simulink model "PID_test_1_hydra"  (R2025b)
settings: Solver=FixedStepAuto  StartTime=0.0  StopTime=inf  RelTol=1e-3  EnableMultiTasking=on
undefined symbols (not defined in the file or in its folder): DiscIntNeverNeededParam
libraries: px4uORBlib x2, px4Sensorslib x2, simulink x1, sharedtransform x1, aerolibutil x1, px4Peripheralslib x1
settings Model: SimulationMode=external  ExtModeTrigDuration=10  Creator=lukas  LastModifiedBy=lukas
settings SolverCC: PositivePriorityOrder=on  AutoInsertRateTranBlk=on
settings OptimizationCC: EnhancedBackFolding=on  PassReuseOutputArgsAs=Individual arguments  ZeroExternalMemoryAtStartup=off  ZeroInternalMemoryAtStartup=off  MaxStackSize=64  OptimizeBlockOrder=speed  DifferentSizesBufferReuse=on  OptimizationCustomize=off  EfficientTunableParamExpr=on
settings DebuggingCC: MultiTaskRateTransMsg=warning  ParameterTunabilityLossMsg=error
settings HardwareCC: ProdBitPerPointer=32.0  ProdBitPerSizeT=32.0  ProdBitPerPtrDiffT=32.0  ProdLargestAtomicInteger=Long  ProdLargestAtomicFloat=Double  ProdWordSize=32.0  ProdLongLongMode=on  ProdHWDeviceType=ARM Compatible->ARM Cortex
settings SFSimCC: MATLABDynamicMemAlloc=off  SimTargetLang=C++  SimDLTargetLibrary=mkl-dnn
settings RTWCC: SystemTargetFile=ert.tlc  HardwareBoard=PX4 Host Target  TLCOptions="-aInlineSetEventsForThisBaseRateFcn=TLC_FALSE -aSuppressMultiTaskScheduler=TLC_FALSE  -aRateBasedStepFcn=0"  TemplateMakefile=ert_default_tmf  Toolchain=GNU Tools for PX4 Autopilots  PortableWordSizes=on  TargetLang=C++  Description=Embedded Coder
settings CodeAppCC: ForceParamTrailComments=on  IgnoreCustomStorageClasses=off  OperatorAnnotations=on  SimulinkDataObjDesc=on  SFDataObjDesc=on  InsertBlockDesc=on
settings ERTTargetCC: ExtModeTransport=2.0  ExtModeStaticAlloc=on  ExtModeMexFile=ext_xcp  ExtModeIntrfLevel=Level2 - Open  InlinedParameterPlacement=Hierarchical

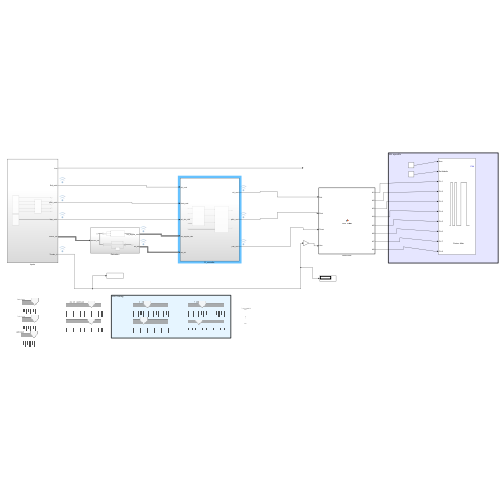
[thumbnail: Simulink's stored preview of the top-level diagram]
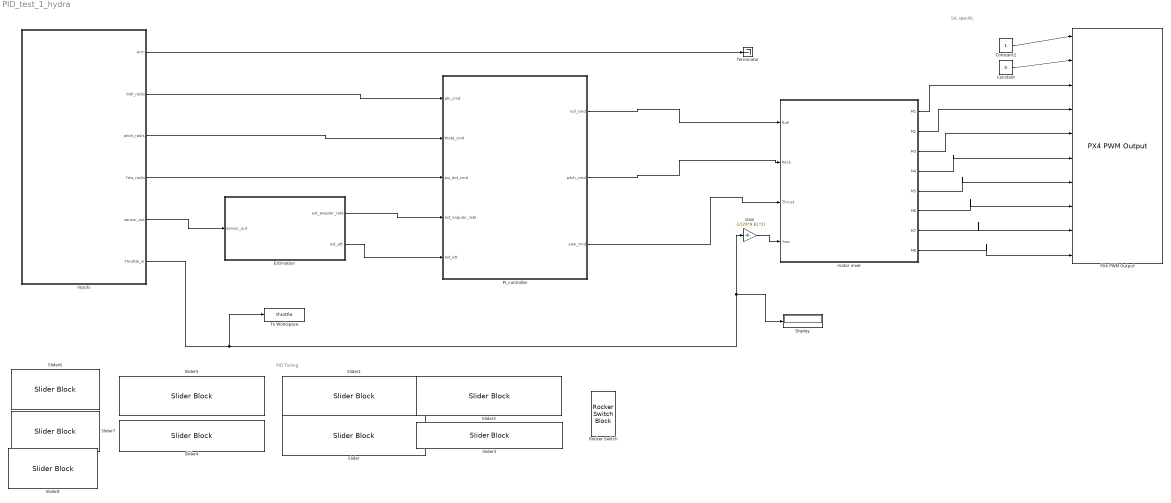
== system PID_test_1_hydra ==
  note: PID Tuning
  note: SIL specific
  Constant : Constant  Value=0  OutDataTypeStr=boolean
  Constant2 : Constant  OutDataTypeStr=boolean
  Display : Display
  Estimation : Subsystem
  Gain : Gain  Gain=-1/(20*9.81*2)
  Inputs : Subsystem
  "PI_controller " : Subsystem
  PX4 PWM Output : px4Peripheralslib/PX4 PWM Output  pwmDevice=Main  pwmChannel1_=on  pwmChannel2_=on  pwmChannel3_=on  pwmChannel4_=on  pwmChannel5_=on  pwmChannel6_=on  pwmChannel7_=on  pwmChannel8_=on
  Rocker Switch : RockerSwitchBlock
  Slider : SliderBlock  ScaleMax=0.1
  Slider1 : SliderBlock  ScaleMax=0.5
  Slider2 : SliderBlock  ScaleMax=0.5
  Slider3 : SliderBlock  ScaleMax=0.1
  Slider4 : SliderBlock  ScaleMax=1
  Slider5 : SliderBlock  ScaleMax=1
  Slider6 : SliderBlock  ScaleMax=4.5
  Slider7 : SliderBlock  ScaleMax=4.5
  Slider8 : SliderBlock  ScaleMax=4.5
  Terminator : Terminator
  To Workspace : ToWorkspace  VariableName=throttle  SaveFormat=Structure With Time  SampleTime=-1
  motor mxer : MATLAB Function  TreatAsAtomicUnit=on
  wires:
  "PI_controller "/2(pitch_cmd) -> motor mxer/2(Pitch)
  motor mxer/5(M5) -> PX4 PWM Output/7
  motor mxer/1(M1) -> PX4 PWM Output/3
  motor mxer/6(M6) -> PX4 PWM Output/8
  motor mxer/7(M7) -> PX4 PWM Output/9
  Constant/1 -> PX4 PWM Output/2
  motor mxer/3(M3) -> PX4 PWM Output/5
  Constant2/1 -> PX4 PWM Output/1
  Gain/1 -> motor mxer/4(Yaw)
  motor mxer/2(M2) -> PX4 PWM Output/4
  "PI_controller "/3(yaw_cmd) -> motor mxer/3(Thrust)
  Inputs/4(Yaw_rad/s) -> "PI_controller "/3(psi_dot_cmd)
  Inputs/1(Arm) -> Terminator/1
  Inputs/2(Roll_rad/s) -> "PI_controller "/1(phi_cmd)
  motor mxer/4(M4) -> PX4 PWM Output/6
  Inputs/6(Throttle_in) -> To Workspace/1, Gain/1, Display/1
  Inputs/3(pitch_rad/s) -> "PI_controller "/2(theta_cmd)
  motor mxer/8(M8) -> PX4 PWM Output/10
  Estimation/2(est_att) -> "PI_controller "/5(est_att)
  Inputs/5(sensor_out) -> Estimation/1(sensor_out)
  Estimation/1(est_angular_rate) -> "PI_controller "/4(est_angular_rate)
  "PI_controller "/1(roll_cmd) -> motor mxer/1(Roll)

== system PID_test_1_hydra/Estimation ==
  sensor_out : Inport
  Bus Creator : BusCreator  Inputs=3
  Bus Selector : BusSelector  OutputSignals=w_x_meas,w_y_meas,w_z_meas
  Bus Selector1 : BusSelector  OutputSignals=roll_meas,pitch_meas,yaw_meas
  MATLAB Function : MATLAB Function  TreatAsAtomicUnit=on
  Subsystem3 : Subsystem
  est_angular_rate : Outport
  est_att : Outport  Port=2
  wires:
  Subsystem3/1(est_angular_rate) -> est_angular_rate/1
  sensor_out/1 -> Bus Selector1/1, Bus Selector/1
  Bus Selector/1 -> Subsystem3/1(In1)  "<w_x_meas>"
  Bus Selector/2 -> Subsystem3/2(In2)  "<w_y_meas>"
  Bus Selector/3 -> Subsystem3/3(In3)  "<w_z_meas>"
  Bus Selector1/1 -> Bus Creator/1  "<roll_meas>"
  Bus Selector1/2 -> Bus Creator/2  "<pitch_meas>"
  Bus Selector1/3 -> MATLAB Function/1(yaw_w)  "<yaw_meas>"
  Bus Creator/1 -> est_att/1
  MATLAB Function/1(yaw_u) -> Bus Creator/3  "yaw"

== system PID_test_1_hydra/Inputs ==
  RC_input : Subsystem
  Sensors_meas : Subsystem
  Stick_mapping : Subsystem
  Arm : Outport
  Roll_rad/s : Outport  Port=2
  pitch_rad/s : Outport  Port=3
  Yaw_rad/s : Outport  Port=4
  sensor_out : Outport  Port=5
  Throttle_in : Outport  Port=6
  wires:
  Sensors_meas/1(sensor_out) -> sensor_out/1
  RC_input/1(Arm) -> Arm/1
  RC_input/2(Roll_in) -> Stick_mapping/1(Roll_in)
  RC_input/3(Pitch_in) -> Stick_mapping/2(Pitch_in)
  RC_input/4(Throttle_in) -> Stick_mapping/3(Throttle_in)
  RC_input/5(Yaw_in) -> Stick_mapping/4(yaw_in)
  Stick_mapping/1(Roll_rad) -> Roll_rad/s/1
  Stick_mapping/2(Pitch_rad) -> pitch_rad/s/1
  Stick_mapping/3(Throttle) -> Throttle_in/1
  Stick_mapping/4(yaw_rad/s) -> Yaw_rad/s/1

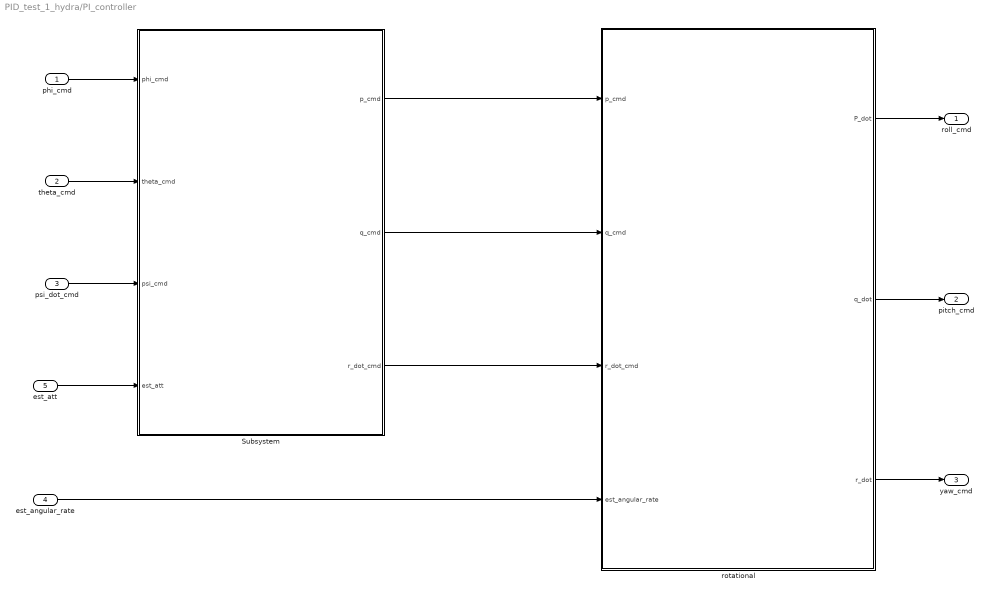
== system PID_test_1_hydra/PI_controller  ==
  phi_cmd : Inport
  theta_cmd : Inport  Port=2
  psi_dot_cmd : Inport  Port=3
  est_angular_rate : Inport  Port=4
  est_att : Inport  Port=5
  Subsystem : Subsystem
  rotational : Subsystem
  roll_cmd : Outport
  pitch_cmd : Outport  Port=2
  yaw_cmd : Outport  Port=3
  wires:
  phi_cmd/1 -> Subsystem/1(phi_cmd)
  theta_cmd/1 -> Subsystem/2(theta_cmd)
  psi_dot_cmd/1 -> Subsystem/3(psi_cmd)
  est_att/1 -> Subsystem/4(est_att)
  est_angular_rate/1 -> rotational/4(est_angular_rate)
  Subsystem/1(p_cmd) -> rotational/1(p_cmd)
  Subsystem/2(q_cmd) -> rotational/2(q_cmd)
  Subsystem/3(r_dot_cmd) -> rotational/3(r_dot_cmd)
  rotational/1(P_dot) -> roll_cmd/1
  rotational/2(q_dot) -> pitch_cmd/1
  rotational/3(r_dot) -> yaw_cmd/1

== system PID_test_1_hydra/Estimation/Subsystem3 ==
  In1 : Inport
  In2 : Inport  Port=2
  In3 : Inport  Port=3
  Bus Creator : BusCreator  Inputs=3
  Subsystem : Subsystem
  Subsystem1 : Subsystem
  Subsystem2 : Subsystem
  est_angular_rate : Outport
  wires:
  Bus Creator/1 -> est_angular_rate/1
  Subsystem/1(Out1) -> Bus Creator/1  "est_p"
  In3/1 -> Subsystem2/1(In1)
  In2/1 -> Subsystem1/1(In1)
  Subsystem2/1(Out1) -> Bus Creator/3  "est_r"
  Subsystem1/1(Out1) -> Bus Creator/2  "est_q"
  In1/1 -> Subsystem/1(In1)

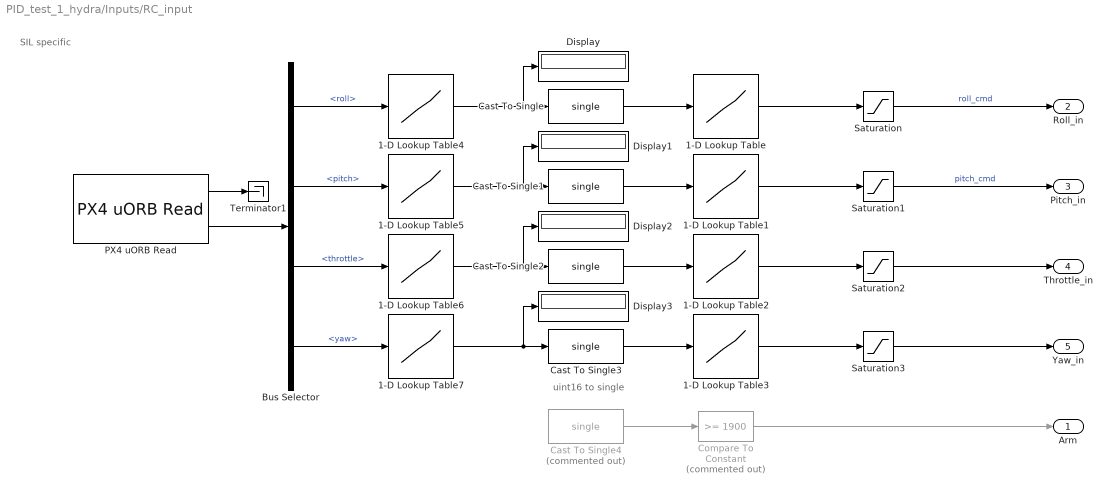
== system PID_test_1_hydra/Inputs/RC_input ==
  note: uint16 to single
  note: SIL specific
  1-D Lookup Table : Lookup_n-D  NumberOfTableDimensions=1  BreakpointsForDimension1=([1000 1500 2000])  Table=single([-1 0 1])  InternalRulePriority=Speed  RndMeth=Simplest
  1-D Lookup Table1 : Lookup_n-D  NumberOfTableDimensions=1  BreakpointsForDimension1=([1000 1500 2000])  Table=single([-1 0 1])  InternalRulePriority=Speed  RndMeth=Simplest
  1-D Lookup Table2 : Lookup_n-D  NumberOfTableDimensions=1  BreakpointsForDimension1=([1000 1500 2000])  Table=single([0 0.5 1])  InternalRulePriority=Speed  RndMeth=Simplest
  1-D Lookup Table3 : Lookup_n-D  NumberOfTableDimensions=1  BreakpointsForDimension1=([1000 1500 2000])  Table=single([-1 0 1])  InternalRulePriority=Speed  RndMeth=Simplest
  1-D Lookup Table4 : Lookup_n-D  NumberOfTableDimensions=1  BreakpointsForDimension1=[-1, 0,1]  Table=single([1000, 1500, 2000])  InternalRulePriority=Speed  RndMeth=Simplest
  1-D Lookup Table5 : Lookup_n-D  NumberOfTableDimensions=1  BreakpointsForDimension1=[-1, 0,1]  Table=single([1000, 1500, 2000])  InternalRulePriority=Speed  RndMeth=Simplest
  1-D Lookup Table6 : Lookup_n-D  NumberOfTableDimensions=1  BreakpointsForDimension1=[0,1]  Table="single([1000,  2000])"  InternalRulePriority=Speed  RndMeth=Simplest
  1-D Lookup Table7 : Lookup_n-D  NumberOfTableDimensions=1  BreakpointsForDimension1=[-1, 0,1]  Table=single([1000, 1500, 2000])  InternalRulePriority=Speed  RndMeth=Simplest
  Bus Selector : BusSelector  OutputSignals=roll,pitch,throttle,yaw
  Cast To Single{,1..3} (4 alike) : DataTypeConversion  OutDataTypeStr=single  SaturateOnIntegerOverflow=off  RndMeth=Floor
  Cast To Single4 : DataTypeConversion  Commented=on  OutDataTypeStr=single  SaturateOnIntegerOverflow=off  RndMeth=Floor
  Compare To Constant : simulink/Logic and Bit Operations/Compare To Constant  Commented=on  relop=>=  const=1900  OutDataTypeStr=boolean
  Display{,1..3} (4 alike) : Display
  PX4 uORB Read : px4uORBlib/PX4 uORB Read  uORBTopic=ManualControlSetpoint  selectInstance=manual_control_setpoint  SampleTime=0.001  BlockingMode=off  BlockTimeout=1e-3
  Saturation : Saturate  UpperLimit=1  LowerLimit=-1
  Saturation1 : Saturate  UpperLimit=1  LowerLimit=-1
  Saturation2 : Saturate  UpperLimit=1  LowerLimit=0
  Saturation3 : Saturate  UpperLimit=1  LowerLimit=-1
  Terminator1 : Terminator
  Arm : Outport
  Roll_in : Outport  Port=2
  Pitch_in : Outport  Port=3
  Throttle_in : Outport  Port=4
  Yaw_in : Outport  Port=5
  wires:
  Compare To Constant/1 -> Arm/1
  Bus Selector/3 -> 1-D Lookup Table6/1  "<throttle>"
  Saturation3/1 -> Yaw_in/1
  Cast To Single/1 -> 1-D Lookup Table/1
  Saturation2/1 -> Throttle_in/1
  Bus Selector/2 -> 1-D Lookup Table5/1  "<pitch>"
  Cast To Single1/1 -> 1-D Lookup Table1/1
  Cast To Single3/1 -> 1-D Lookup Table3/1
  Cast To Single4/1 -> Compare To Constant/1
  Cast To Single2/1 -> 1-D Lookup Table2/1
  Saturation1/1 -> Pitch_in/1  "pitch_cmd"
  Saturation/1 -> Roll_in/1  "roll_cmd"
  1-D Lookup Table/1 -> Saturation/1
  1-D Lookup Table1/1 -> Saturation1/1
  1-D Lookup Table2/1 -> Saturation2/1
  1-D Lookup Table3/1 -> Saturation3/1
  Bus Selector/4 -> 1-D Lookup Table7/1  "<yaw>"
  Bus Selector/1 -> 1-D Lookup Table4/1  "<roll>"
  PX4 uORB Read/2 -> Bus Selector/1
  PX4 uORB Read/1 -> Terminator1/1
  1-D Lookup Table4/1 -> Display/1, Cast To Single/1
  1-D Lookup Table5/1 -> Display1/1, Cast To Single1/1
  1-D Lookup Table7/1 -> Display3/1, Cast To Single3/1
  1-D Lookup Table6/1 -> Display2/1, Cast To Single2/1

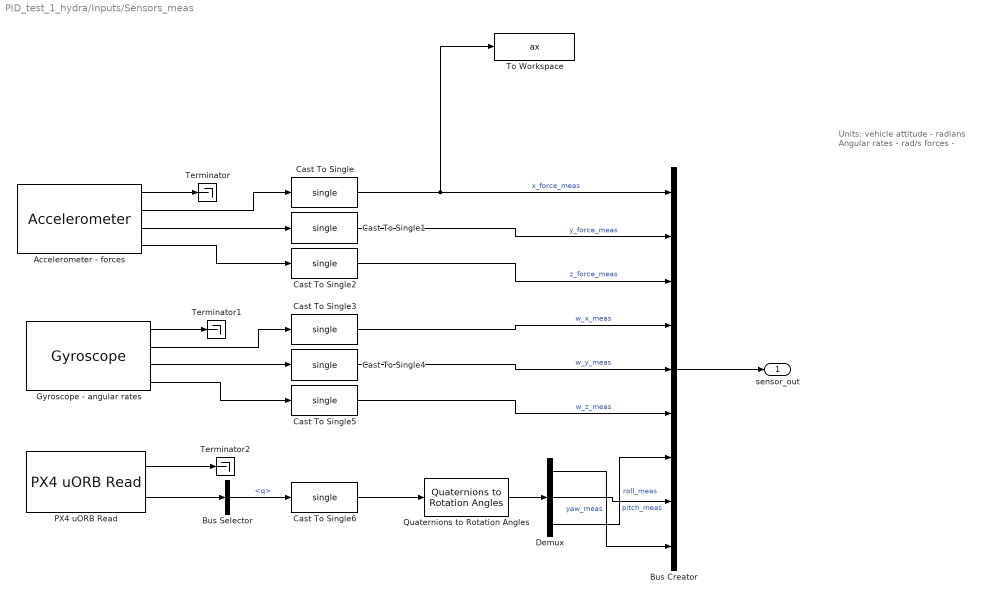
== system PID_test_1_hydra/Inputs/Sensors_meas ==
  note: Units:
      | vehicle attitude - radians
      | Angular rates - rad/s
      | forces -
  "Accelerometer - forces " : px4Sensorslib/Accelerometer  uorbTimeStamp=off  BlockingMode=off  BlockTimeout=1e-3  sampleTime=1/250
  Bus Creator : BusCreator  Inputs=9
  Bus Selector : BusSelector  OutputSignals=q
  Cast To Single{,1..6} (7 alike) : DataTypeConversion  OutDataTypeStr=single  SaturateOnIntegerOverflow=off  RndMeth=Floor
  Demux : Demux  Outputs=3
  Gyroscope - angular rates : px4Sensorslib/Gyroscope  uorbTimeStamp=off  BlockingMode=off  BlockTimeout=1e-3  sampleTime=1/250
  PX4 uORB Read : px4uORBlib/PX4 uORB Read  uORBTopic=VehicleAttitude  selectInstance=vehicle_attitude  SampleTime=-1  BlockingMode=off  BlockTimeout=1e-3
  Quaternions to Rotation Angles : sharedtransform/Quaternions to Rotation Angles  rotationOrder=ZYX  aMode=aMode
  Terminator : Terminator
  Terminator1 : Terminator
  Terminator2 : Terminator
  To Workspace : ToWorkspace  VariableName=ax  SaveFormat=Structure With Time  SampleTime=-1
  sensor_out : Outport
  wires:
  PX4 uORB Read/1 -> Terminator2/1
  Gyroscope - angular rates/1 -> Terminator1/1
  Cast To Single4/1 -> Bus Creator/5  "w_y_meas"
  Gyroscope - angular rates/2 -> Cast To Single3/1
  "Accelerometer - forces "/1 -> Terminator/1
  Demux/3 -> Bus Creator/7  "roll_meas"
  Demux/2 -> Bus Creator/8  "pitch_meas"
  Demux/1 -> Bus Creator/9  "yaw_meas"
  Gyroscope - angular rates/3 -> Cast To Single4/1
  Gyroscope - angular rates/4 -> Cast To Single5/1
  Cast To Single5/1 -> Bus Creator/6  "w_z_meas"
  Bus Creator/1 -> sensor_out/1
  "Accelerometer - forces "/2 -> Cast To Single/1
  Bus Selector/1 -> Cast To Single6/1  "<q>"
  "Accelerometer - forces "/3 -> Cast To Single1/1
  Cast To Single/1 -> To Workspace/1, Bus Creator/1  "x_force_meas"
  PX4 uORB Read/2 -> Bus Selector/1
  "Accelerometer - forces "/4 -> Cast To Single2/1
  Cast To Single6/1 -> Quaternions to Rotation Angles/1
  Quaternions to Rotation Angles/1 -> Demux/1
  Cast To Single3/1 -> Bus Creator/4  "w_x_meas"
  Cast To Single1/1 -> Bus Creator/2  "y_force_meas"
  Cast To Single2/1 -> Bus Creator/3  "z_force_meas"

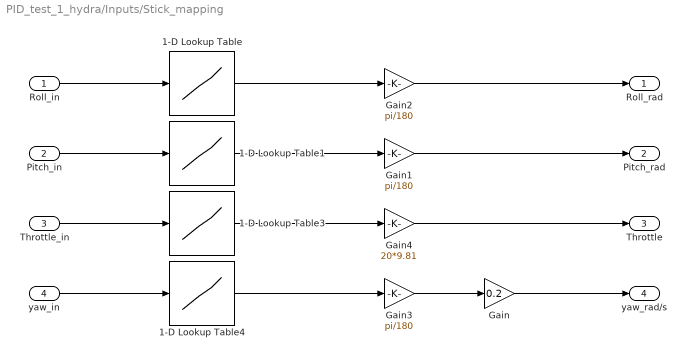
== system PID_test_1_hydra/Inputs/Stick_mapping ==
  Roll_in : Inport
  Pitch_in : Inport  Port=2
  Throttle_in : Inport  Port=3
  yaw_in : Inport  Port=4
  1-D Lookup Table : Lookup_n-D  NumberOfTableDimensions=1  BreakpointsForDimension1=single([-1,1])  Table=single([-30,30])  InternalRulePriority=Speed  RndMeth=Simplest
  1-D Lookup Table1 : Lookup_n-D  NumberOfTableDimensions=1  BreakpointsForDimension1=single([-1,1])  Table=single([30,-30])  InternalRulePriority=Speed  RndMeth=Simplest
  1-D Lookup Table3 : Lookup_n-D  NumberOfTableDimensions=1  BreakpointsForDimension1=single([0 0.100000001 0.25 0.5 0.75 1])  Table=single([0 -0.200000003 -0.5 -1 -1.5 -2])  InternalRulePriority=Speed  RndMeth=Simplest
  1-D Lookup Table4 : Lookup_n-D  NumberOfTableDimensions=1  BreakpointsForDimension1=single([-1,1])  Table=single([-90,90])  InternalRulePriority=Speed  RndMeth=Simplest
  Gain : Gain  Gain=0.2
  Gain1 : Gain  Gain=pi/180
  Gain2 : Gain  Gain=pi/180
  Gain3 : Gain  Gain=pi/180
  Gain4 : Gain  Gain=20*9.81
  Roll_rad : Outport
  Pitch_rad : Outport  Port=2
  Throttle : Outport  Port=3
  yaw_rad/s : Outport  Port=4
  wires:
  Gain1/1 -> Pitch_rad/1
  Roll_in/1 -> 1-D Lookup Table/1
  Pitch_in/1 -> 1-D Lookup Table1/1
  yaw_in/1 -> 1-D Lookup Table4/1
  Throttle_in/1 -> 1-D Lookup Table3/1
  1-D Lookup Table1/1 -> Gain1/1
  1-D Lookup Table/1 -> Gain2/1
  1-D Lookup Table3/1 -> Gain4/1
  1-D Lookup Table4/1 -> Gain3/1
  Gain2/1 -> Roll_rad/1
  Gain3/1 -> Gain/1
  Gain4/1 -> Throttle/1
  Gain/1 -> yaw_rad/s/1

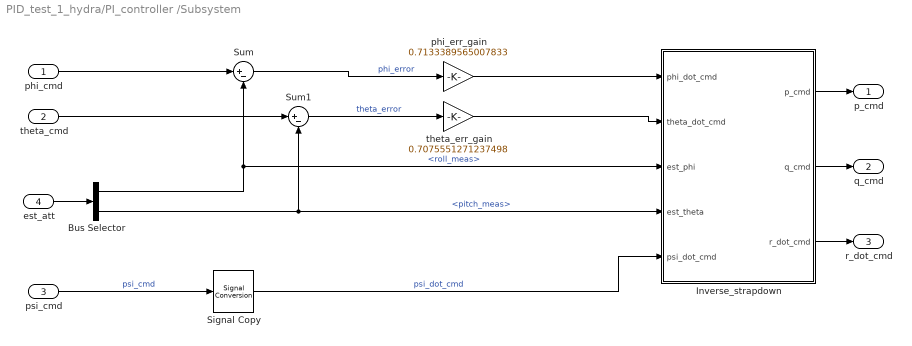
== system PID_test_1_hydra/PI_controller /Subsystem ==
  phi_cmd : Inport
  theta_cmd : Inport  Port=2
  psi_cmd : Inport  Port=3
  est_att : Inport  Port=4
  Bus Selector : BusSelector  OutputSignals=roll_meas,pitch_meas
  Inverse_strapdown : Subsystem
  Signal Copy : SignalConversion  OverrideOpt=off
  Sum : Sum  Inputs=|+-
  Sum1 : Sum  Inputs=|+-
  phi_err_gain : Gain  Gain=0.7133389565007833
  theta_err_gain : Gain  Gain=0.7075551271237498
  p_cmd : Outport
  q_cmd : Outport  Port=2
  r_dot_cmd : Outport  Port=3
  wires:
  Bus Selector/2 -> Inverse_strapdown/4(est_theta), Sum1/2  "<pitch_meas>"
  Bus Selector/1 -> Inverse_strapdown/3(est_phi), Sum/2  "<roll_meas>"
  Sum1/1 -> theta_err_gain/1  "theta_error"
  theta_cmd/1 -> Sum1/1
  phi_cmd/1 -> Sum/1
  Sum/1 -> phi_err_gain/1  "phi_error"
  psi_cmd/1 -> Signal Copy/1  "psi_cmd"
  Signal Copy/1 -> Inverse_strapdown/5(psi_dot_cmd)  "psi_dot_cmd"
  est_att/1 -> Bus Selector/1
  phi_err_gain/1 -> Inverse_strapdown/1(phi_dot_cmd)
  theta_err_gain/1 -> Inverse_strapdown/2(theta_dot_cmd)
  Inverse_strapdown/1(p_cmd) -> p_cmd/1
  Inverse_strapdown/2(q_cmd) -> q_cmd/1
  Inverse_strapdown/3(r_dot_cmd) -> r_dot_cmd/1

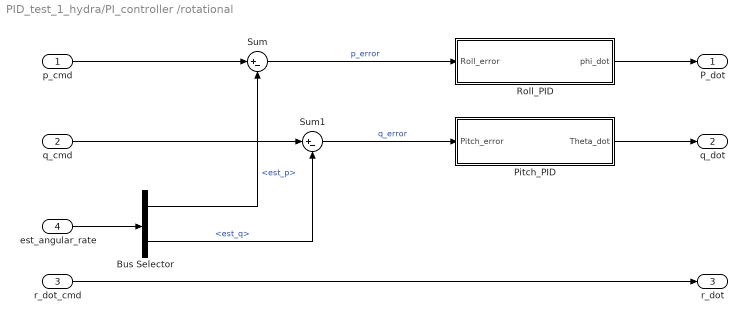
== system PID_test_1_hydra/PI_controller /rotational ==
  p_cmd : Inport
  q_cmd : Inport  Port=2
  r_dot_cmd : Inport  Port=3
  est_angular_rate : Inport  Port=4
  Bus Selector : BusSelector  OutputSignals=est_p,est_q
  Pitch_PID : Subsystem
  Roll_PID : Subsystem
  Sum : Sum  Inputs=|+-
  Sum1 : Sum  Inputs=|+-
  P_dot : Outport
  q_dot : Outport  Port=2
  r_dot : Outport  Port=3
  wires:
  Sum/1 -> Roll_PID/1(Roll_error)  "p_error"
  Sum1/1 -> Pitch_PID/1(Pitch_error)  "q_error"
  Roll_PID/1(phi_dot) -> P_dot/1
  Bus Selector/2 -> Sum1/2  "<est_q>"
  p_cmd/1 -> Sum/1
  Pitch_PID/1(Theta_dot) -> q_dot/1
  r_dot_cmd/1 -> r_dot/1
  q_cmd/1 -> Sum1/1
  Bus Selector/1 -> Sum/2  "<est_p>"
  est_angular_rate/1 -> Bus Selector/1

== system PID_test_1_hydra/Estimation/Subsystem3/Subsystem ==
  In1 : Inport
  DI : Subsystem
  Gain : Gain  Gain=single(4.5)
  Saturation1 : Saturate  UpperLimit=5.24  LowerLimit=-5.24
  Sum : Sum  Inputs=|+-
  Out1 : Outport
  wires:
  Sum/1 -> Gain/1
  Gain/1 -> DI/1(In1)
  DI/1(Out1) -> Saturation1/1, Sum/2
  In1/1 -> DI/2(In2), Sum/1
  Saturation1/1 -> Out1/1

== system PID_test_1_hydra/Estimation/Subsystem3/Subsystem1 ==
  In1 : Inport
  DI : Subsystem
  Gain : Gain  Gain=4.5
  Saturation1 : Saturate  UpperLimit=5.24  LowerLimit=-5.24
  Sum : Sum  Inputs=|+-
  Out1 : Outport
  wires:
  Sum/1 -> Gain/1
  DI/1(Out1) -> Saturation1/1, Sum/2
  Gain/1 -> DI/1(In1)
  In1/1 -> DI/2(In2), Sum/1
  Saturation1/1 -> Out1/1

== system PID_test_1_hydra/Estimation/Subsystem3/Subsystem2 ==
  In1 : Inport
  DI : Subsystem
  Gain : Gain  Gain=4.5
  Saturation1 : Saturate  UpperLimit=5.24  LowerLimit=-5.24
  Sum : Sum  Inputs=|+-
  Out1 : Outport
  wires:
  Sum/1 -> Gain/1
  DI/1(Out1) -> Saturation1/1, Sum/2
  Gain/1 -> DI/1(In1)
  In1/1 -> DI/2(In2), Sum/1
  Saturation1/1 -> Out1/1

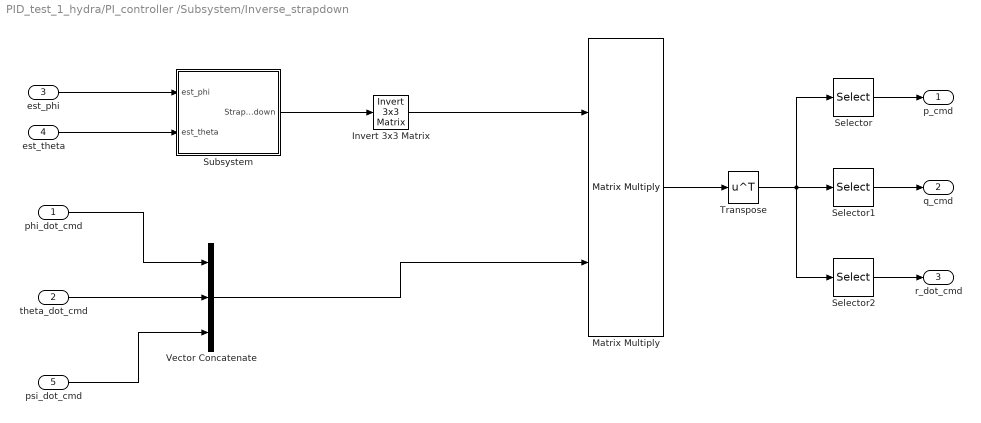
== system PID_test_1_hydra/PI_controller /Subsystem/Inverse_strapdown ==
  phi_dot_cmd : Inport
  theta_dot_cmd : Inport  Port=2
  est_phi : Inport  Port=3
  est_theta : Inport  Port=4
  psi_dot_cmd : Inport  Port=5
  Invert 3x3 Matrix : aerolibutil/Invert  3x3 Matrix
  Matrix Multiply : Product  Multiplication=Matrix(*)
  Selector : Selector  InputPortWidth=3  IndexOptions=Index vector (dialog)  Indices=1  OutputSizes=1
  Selector1 : Selector  InputPortWidth=3  IndexOptions=Index vector (dialog)  Indices=2  OutputSizes=1
  Selector2 : Selector  InputPortWidth=3  IndexOptions=Index vector (dialog)  Indices=3  OutputSizes=1
  Subsystem : Subsystem
  Transpose : Math  Operator=transpose
  Vector Concatenate : Concatenate  NumInputs=3  Mode=Multidimensional array
  p_cmd : Outport
  q_cmd : Outport  Port=2
  r_dot_cmd : Outport  Port=3
  wires:
  Vector Concatenate/1 -> Matrix Multiply/2
  Subsystem/1(Strap_down) -> Invert 3x3 Matrix/1
  Invert 3x3 Matrix/1 -> Matrix Multiply/1
  est_phi/1 -> Subsystem/1(est_phi)
  est_theta/1 -> Subsystem/2(est_theta)
  Matrix Multiply/1 -> Transpose/1
  Transpose/1 -> Selector2/1, Selector1/1, Selector/1
  Selector/1 -> p_cmd/1
  Selector1/1 -> q_cmd/1
  Selector2/1 -> r_dot_cmd/1
  phi_dot_cmd/1 -> Vector Concatenate/1
  theta_dot_cmd/1 -> Vector Concatenate/2
  psi_dot_cmd/1 -> Vector Concatenate/3

== system PID_test_1_hydra/PI_controller /rotational/Pitch_PID ==
  Pitch_error : Inport
  Discrete-Time Integrator : DiscreteIntegrator  SampleTime=-1  ICPrevOutput=DiscIntNeverNeededParam  ICPrevScaledInput=DiscIntNeverNeededParam
  I_pitch : Gain  Gain=single(0.02936526)
  P_pitch : Gain  Gain=0.2
  Sum : Sum  Inputs=|++
  Theta_dot : Outport
  wires:
  Sum/1 -> Theta_dot/1
  Discrete-Time Integrator/1 -> I_pitch/1
  P_pitch/1 -> Sum/1
  Pitch_error/1 -> Discrete-Time Integrator/1, P_pitch/1
  I_pitch/1 -> Sum/2

== system PID_test_1_hydra/PI_controller /rotational/Roll_PID ==
  Roll_error : Inport
  Discrete-Time Integrator : DiscreteIntegrator  gainval=1  SampleTime=-1  ICPrevOutput=DiscIntNeverNeededParam  ICPrevScaledInput=DiscIntNeverNeededParam
  I_roll : Gain  Gain=0.03033785294146734
  P_roll : Gain  Gain=0.2
  Sum : Sum  Inputs=|++
  phi_dot : Outport
  wires:
  Sum/1 -> phi_dot/1
  P_roll/1 -> Sum/1
  I_roll/1 -> Discrete-Time Integrator/1  "int_err_unsat"
  Discrete-Time Integrator/1 -> Sum/2
  Roll_error/1 -> I_roll/1, P_roll/1

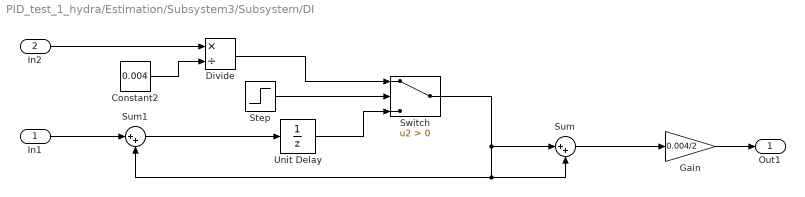
== system PID_test_1_hydra/Estimation/Subsystem3/Subsystem/DI ==
  In1 : Inport
  In2 : Inport  Port=2
  Constant2 : Constant  Value=0.004
  Divide : Product  Inputs=*/
  Gain : Gain  Gain=0.004/2
  Step : Step  Time=0.02  Before=1  After=0  SampleTime=0.004
  Sum : Sum  Inputs=|++
  Sum1 : Sum  Inputs=|++
  Switch : Switch  Criteria=u2 > Threshold  SaturateOnIntegerOverflow=off  InputSameDT=off
  Unit Delay : UnitDelay  SampleTime=-1  HasFrameUpgradeWarning=on
  Out1 : Outport
  wires:
  Step/1 -> Switch/2
  Sum1/1 -> Unit Delay/1
  Unit Delay/1 -> Switch/3
  Divide/1 -> Switch/1
  Switch/1 -> Sum1/2, Sum/2, Sum/1
  Sum/1 -> Gain/1
  Constant2/1 -> Divide/2
  Gain/1 -> Out1/1
  In1/1 -> Sum1/1
  In2/1 -> Divide/1

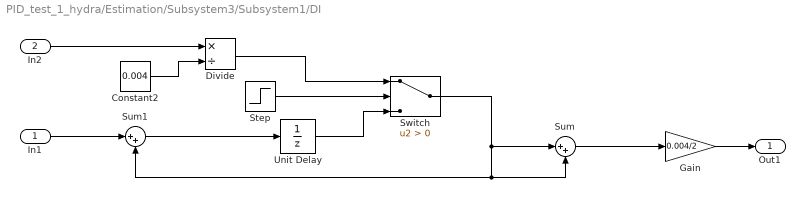
== system PID_test_1_hydra/Estimation/Subsystem3/Subsystem1/DI ==
  In1 : Inport
  In2 : Inport  Port=2
  Constant2 : Constant  Value=0.004
  Divide : Product  Inputs=*/
  Gain : Gain  Gain=0.004/2
  Step : Step  Time=0.02  Before=1  After=0  SampleTime=0.004
  Sum : Sum  Inputs=|++
  Sum1 : Sum  Inputs=|++
  Switch : Switch  Criteria=u2 > Threshold  SaturateOnIntegerOverflow=off  InputSameDT=off
  Unit Delay : UnitDelay  SampleTime=-1  HasFrameUpgradeWarning=on
  Out1 : Outport
  wires:
  Step/1 -> Switch/2
  Sum1/1 -> Unit Delay/1
  Unit Delay/1 -> Switch/3
  Divide/1 -> Switch/1
  Switch/1 -> Sum1/2, Sum/2, Sum/1
  Sum/1 -> Gain/1
  Constant2/1 -> Divide/2
  Gain/1 -> Out1/1
  In1/1 -> Sum1/1
  In2/1 -> Divide/1

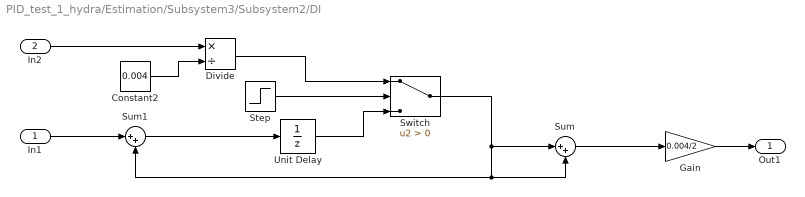
== system PID_test_1_hydra/Estimation/Subsystem3/Subsystem2/DI ==
  In1 : Inport
  In2 : Inport  Port=2
  Constant2 : Constant  Value=0.004
  Divide : Product  Inputs=*/
  Gain : Gain  Gain=0.004/2
  Step : Step  Time=0.02  Before=1  After=0  SampleTime=0.004
  Sum : Sum  Inputs=|++
  Sum1 : Sum  Inputs=|++
  Switch : Switch  Criteria=u2 > Threshold  SaturateOnIntegerOverflow=off  InputSameDT=off
  Unit Delay : UnitDelay  SampleTime=-1  HasFrameUpgradeWarning=on
  Out1 : Outport
  wires:
  Step/1 -> Switch/2
  Sum1/1 -> Unit Delay/1
  Unit Delay/1 -> Switch/3
  Divide/1 -> Switch/1
  Switch/1 -> Sum1/2, Sum/2, Sum/1
  Sum/1 -> Gain/1
  Constant2/1 -> Divide/2
  Gain/1 -> Out1/1
  In1/1 -> Sum1/1
  In2/1 -> Divide/1

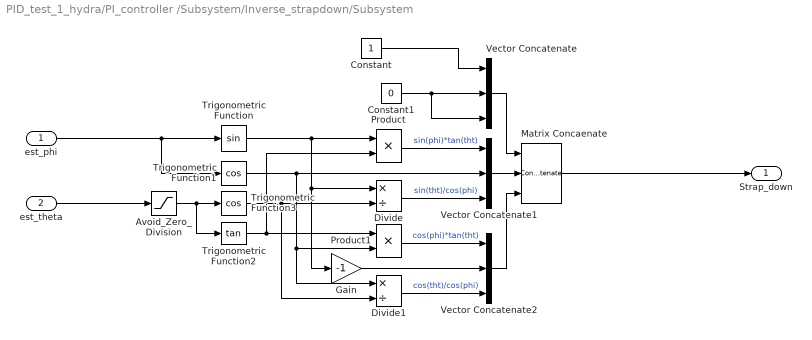
== system PID_test_1_hydra/PI_controller /Subsystem/Inverse_strapdown/Subsystem ==
  est_phi : Inport
  est_theta : Inport  Port=2
  Avoid_Zero_Division : Saturate  UpperLimit=pi/2*0.9  LowerLimit=-pi/2*0.9
  Constant : Constant  OutDataTypeStr=single
  Constant1 : Constant  Value=0  OutDataTypeStr=single
  Divide : Product  Inputs=*/
  Divide1 : Product  Inputs=*/
  Gain : Gain  Gain=-1
  Matrix Concaenate : Concatenate  NumInputs=3  Mode=Multidimensional array  ConcatenateDimension=2
  Product : Product  RndMeth=Zero
  Product1 : Product  RndMeth=Zero
  Trigonometric Function : Trigonometry
  Trigonometric Function1 : Trigonometry  Operator=cos
  Trigonometric Function2 : Trigonometry  Operator=tan
  Trigonometric Function3 : Trigonometry  Operator=cos
  Vector Concatenate : Concatenate  NumInputs=3  Mode=Multidimensional array
  Vector Concatenate1 : Concatenate  NumInputs=3  Mode=Multidimensional array
  Vector Concatenate2 : Concatenate  NumInputs=3  Mode=Multidimensional array
  Strap_down : Outport
  wires:
  Vector Concatenate1/1 -> Matrix Concaenate/2
  Product1/1 -> Vector Concatenate2/1  "cos(phi)*tan(tht)"
  Trigonometric Function1/1 -> Vector Concatenate1/2, Divide1/1, Product1/2
  est_phi/1 -> Trigonometric Function1/1, Trigonometric Function/1
  Constant1/1 -> Vector Concatenate/2, Vector Concatenate/3
  Trigonometric Function3/1 -> Divide/2, Divide1/2
  Avoid_Zero_Division/1 -> Trigonometric Function3/1, Trigonometric Function2/1
  Gain/1 -> Vector Concatenate2/2
  Divide/1 -> Vector Concatenate1/3  "sin(tht)/cos(phi)"
  Vector Concatenate2/1 -> Matrix Concaenate/3
  Divide1/1 -> Vector Concatenate2/3  "cos(tht)/cos(phi)"
  est_theta/1 -> Avoid_Zero_Division/1
  Product/1 -> Vector Concatenate1/1  "sin(phi)*tan(tht)"
  Vector Concatenate/1 -> Matrix Concaenate/1
  Constant/1 -> Vector Concatenate/1
  Matrix Concaenate/1 -> Strap_down/1
  Trigonometric Function2/1 -> Product/2, Product1/1
  Trigonometric Function/1 -> Product/1, Divide/1, Gain/1

== matlab function PID_test_1_hydra/motor mxer ==
  data: Roll input; M1 output; Pitch input; Thrust input; Yaw input; M2 output; M3 output; M4 output; M5 output; M6 output; M7 output; M8 output
function [M1, M2, M3, M4, M5, M6, M7, M8] = motor_mixer(Roll, Pitch, Thrust, Yaw)
% This function calculates motor commands for the 8-motor "plus" 
% configuration shown in your image.
%
% Inputs (assumed):
%   Roll, Pitch, Yaw: -1.0 to +1.0 control inputs
%   Thrust:             0.0 to 1.0 base throttle

% --- Configuration ---
idle_PWM = uint16(1000);
max_motor_val = single(1.0); % Max normalized output
min_motor_val = single(0.0); % Min normalized output

% This scaling method is from your example. It scales the control 
% inputs by the thrust level. You may need to tune the '4.0'
% denominator for best performance.
control_scale = Thrust / single(4.0);

% --- Mixer Logic ---
% Calculate normalized motor values (0.0 to 1.0 range) based on the diagram.
% We use single() to ensure floating-point math, as in your example.

% M1 (Front, CCW): -Pitch, +Yaw
m1_norm = ( ( -Pitch + Yaw ) * control_scale + Thrust );

% M2 (Back, CCW): +Pitch, +Yaw
m2_norm = ( (  Pitch + Yaw ) * control_scale + Thrust );

% M3 (Front-Right, CW): -Pitch, -Roll, -Yaw
m3_norm = ( ( -Pitch - Roll - Yaw ) * control_scale + Thrust );

% M4 (Back-Right, CW): +Pitch, -Roll, -Yaw
m4_norm = ( (  Pitch - Roll - Yaw ) * control_scale + Thrust );

% M5 (Front-Left, CW): -Pitch, +Roll, -Yaw
m5_norm = ( ( -Pitch + Roll - Yaw ) * control_scale + Thrust );

% M6 (Back-Left, CW): +Pitch, +Roll, -Yaw
m6_norm = ( (  Pitch + Roll - Yaw ) * control_scale + Thrust );

% M7 (Left, CCW): +Roll, +Yaw
m7_norm = ( (  Roll + Yaw ) * control_scale + Thrust );

% M8 (Right, CCW): -Roll, +Yaw
m8_norm = ( ( -Roll + Yaw ) * control_scale + Thrust );


% --- Output Scaling and Clamping ---
% It's CRITICAL to clamp (saturate) the motor commands between 0.0 and 1.0
% to prevent errors and ensure motor outputs are valid.
motors_norm = [m1_norm, m2_norm, m3_norm, m4_norm, m5_norm, m6_norm, m7_norm, m8_norm];
motors_norm = min(max(motors_norm, min_motor_val), max_motor_val);

% Convert normalized values (0.0-1.0) to PWM (1000-2000)
M1 = uint16(motors_norm(1) * single(1000)) + idle_PWM;
M2 = uint16(motors_norm(2) * single(1000)) + idle_PWM;
M3 = uint16(motors_norm(3) * single(1000)) + idle_PWM;
M4 = uint16(motors_norm(4) * single(1000)) + idle_PWM;
M5 = uint16(motors_norm(5) * single(1000)) + idle_PWM;
M6 = uint16(motors_norm(6) * single(1000)) + idle_PWM;
M7 = uint16(motors_norm(7) * single(1000)) + idle_PWM;
M8 = uint16(motors_norm(8) * single(1000)) + idle_PWM;

end

== matlab function PID_test_1_hydra/Estimation/MATLAB Function ==
  data: yaw_w input; yaw_u output
function yaw_u = unwrap_yaw(yaw_w)
% yaw_w: wrapped yaw [rad], typically in [-pi, pi]
% yaw_u: continuous yaw [rad]

persistent yaw_prev yaw_accum initialized

if isempty(initialized)
    yaw_prev = yaw_w;
    yaw_accum = yaw_w;
    initialized = true;
end

dyaw = yaw_w - yaw_prev;

% wrap increment to [-pi, pi]
dyaw = mod(dyaw + pi, 2*pi) - pi;

yaw_accum = yaw_accum + dyaw;
yaw_prev = yaw_w;

yaw_u = yaw_accum;
